simulink model "fir_dbl_tap_test"  (Simulink 7.0)
settings: Solver=VariableStepDiscrete  StartTime=0.0  StopTime=50  RelTol=1e-3
libraries: xbsIndex_r4 x8, casper_library x1
settings Model: Creator=User  LastModifiedBy=User
settings DebuggingCC: SaveWithDisabledLinksMsg=none  SaveWithParameterizedLinksMsg=none

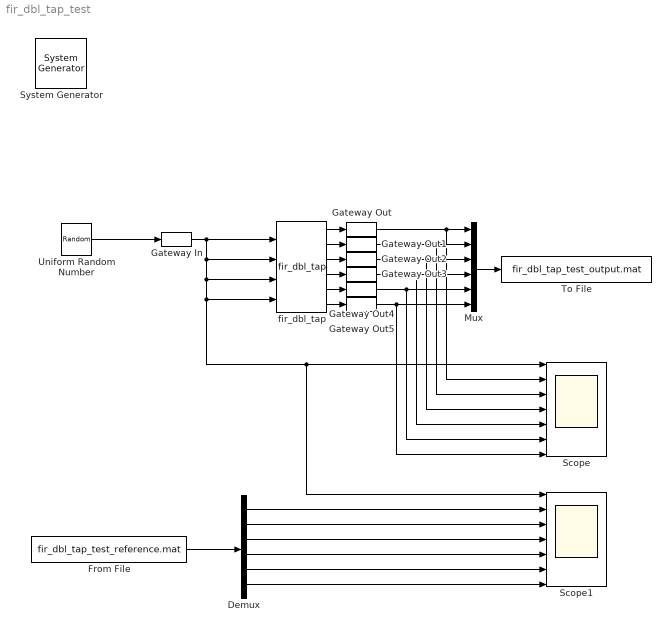
== system fir_dbl_tap_test ==
  " System Generator" : xbsIndex_r4/ System Generator  Tag=genX  SystemSampleTime=-1  xilinxfamily=Virtex4  part=xc4vsx35  speed=-10  package=ff668  synthesis_tool=XST  clock_wrapper=Clock Enables  directory=./netlist  testbench=off  simulink_period=1  sysclk_period=100  dcm_input_clock_period=100  incr_netlist=off  trim_vbits=Everywhere in SubSystem  dbl_ovrd=According to Block Masks  core_generation=According to Block Masks  run_coregen=off  deprecated_control=off  eval_field=0  block_type=sysgen
      settings: block_version=10.1.1
  Demux : Demux  Outputs=6
  From File : FromFile  FileName=fir_dbl_tap_test_reference.mat  SampleTime=1
  Gateway In : xbsIndex_r4/Gateway In  arith_type="Signed  (2's comp)"  n_bits=16  bin_pt=15  quantization=Truncate  overflow=Wrap  period=1  dbl_ovrd=off  timing_constraint=None  locs_specified=off  LOCs={}  block_type=gatewayin
      settings: infoedit="Gateway in block.  Converts inputs of type Simulink integer, double and fixed point to  Xilinx fixed point type.<P><P>Hardware notes:  In hardware these blocks become top level input ports."  block_version=10.1.1
  Gateway Out{,1..5} (6 alike) : xbsIndex_r4/Gateway Out  hdl_port=on  timing_constraint=None  locs_specified=off  LOCs={}  block_type=gatewayout
      settings: infoedit="Gateway out block.  Converts Xilinx fixed point inputs into ouputs of type Simulink integer, double, or fixed point.<P><P>Hardware notes:  In hardware these blocks become top level output ports or are discarded, depending on how they are configured."  block_version=10.1.1
  Mux : Mux  Inputs=6
  Scope : Scope  NumInputPorts=7
      settings: YMin=-5~-5~-5~-5~-5~-5~-5  YMax=5~5~5~5~5~5~5
  Scope1 : Scope  NumInputPorts=7
      settings: YMin=-5~-5~-5~-5~-5~-5~-5  YMax=5~5~5~5~5~5~5
  To File : ToFile  Filename=fir_dbl_tap_test_output.mat  MatrixName=output
  Uniform Random Number : UniformRandomNumber  SampleTime=1
  fir_dbl_tap : casper_library/Downconverter/fir_dbl_tap  SystemSampleTime=-1  factor=0.1234  add_latency=3  mult_latency=4
  wires:
  Uniform Random Number/1 -> Gateway In/1
  Gateway In/1 -> fir_dbl_tap/1, fir_dbl_tap/2, fir_dbl_tap/3, fir_dbl_tap/4, Scope/1, Scope1/1
  fir_dbl_tap/1 -> Gateway Out/1
  fir_dbl_tap/2 -> Gateway Out1/1
  fir_dbl_tap/3 -> Gateway Out2/1
  fir_dbl_tap/4 -> Gateway Out3/1
  fir_dbl_tap/5 -> Gateway Out4/1
  fir_dbl_tap/6 -> Gateway Out5/1
  Gateway Out/1 -> Mux/1, Scope/2
  Gateway Out1/1 -> Mux/2, Scope/3
  Gateway Out2/1 -> Mux/3, Scope/4
  Gateway Out3/1 -> Mux/4, Scope/5
  Gateway Out4/1 -> Mux/5, Scope/6
  Gateway Out5/1 -> Mux/6, Scope/7
  Mux/1 -> To File/1
  From File/1 -> Demux/1
  Demux/1 -> Scope1/2
  Demux/2 -> Scope1/3
  Demux/3 -> Scope1/4
  Demux/4 -> Scope1/5
  Demux/5 -> Scope1/6
  Demux/6 -> Scope1/7
